simulink library "LIB_RespiratorSupervisor"  (R2018b)
settings: Solver=VariableStepAuto  StartTime=0.0  StopTime=10.0  RelTol=1e-3
undefined symbols (not defined in the file or in its folder): eSupervisorStates, tDelayMaxForRespiratorInit, tDelayMaxForTestMode, tMaxDebounceForCycleStop, tMinDebounceForTestStart
libraries: simulink x8, LIB_CycleControl x1
settings Model: Creator=BRAUL  LastModifiedBy=VITIE

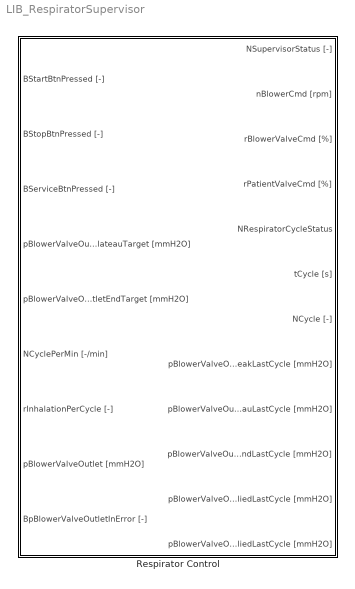
== system LIB_RespiratorSupervisor ==
  Respirator Control : Subsystem
      settings: AttributesFormatString=%<ReferenceBlock>

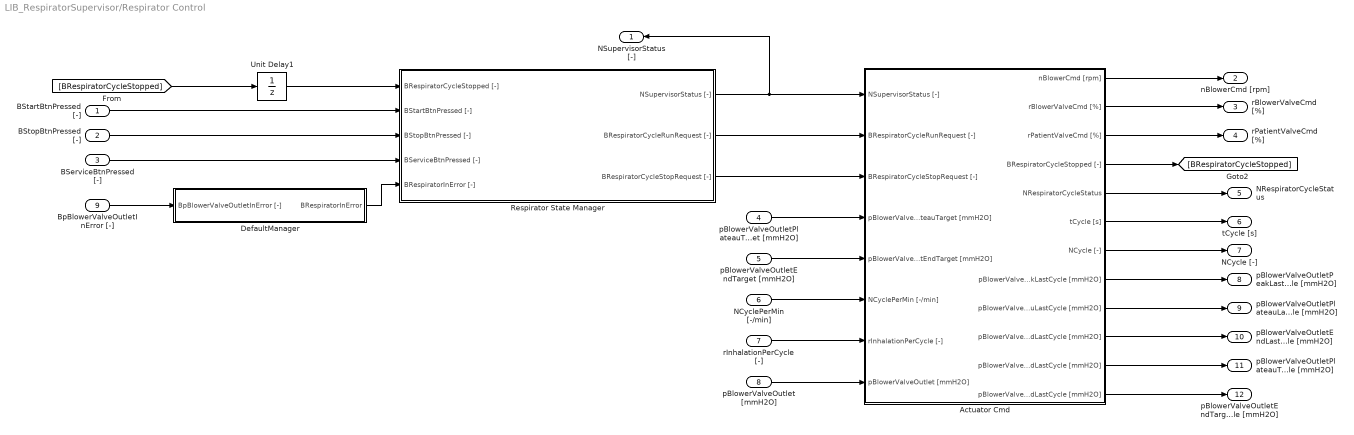
== system LIB_RespiratorSupervisor/Respirator Control ==
  BStartBtnPressed [-] : Inport  OutDataTypeStr=boolean
  BStopBtnPressed [-] : Inport  Port=2  OutDataTypeStr=boolean
  BServiceBtnPressed [-] : Inport  Port=3  OutDataTypeStr=boolean
  pBlowerValveOutletPlateauTarget [mmH2O] : Inport  Port=4  OutDataTypeStr=single
  pBlowerValveOutletEndTarget [mmH2O] : Inport  Port=5  OutDataTypeStr=single
  NCyclePerMin [-/min] : Inport  Port=6  OutDataTypeStr=single
  rInhalationPerCycle [-] : Inport  Port=7  OutDataTypeStr=single
  pBlowerValveOutlet [mmH2O] : Inport  Port=8  OutDataTypeStr=single
  BpBlowerValveOutletInError [-] : Inport  Port=9  OutDataTypeStr=boolean
  Actuator Cmd : Subsystem
  DefaultManager : Subsystem
  Respirator State Manager : Subsystem
  Unit Delay1 : UnitDelay  InitialCondition=false  SampleTime=-1
      settings: AttributesFormatString=%<InitialCondition>
  NSupervisorStatus [-] : Outport  OutDataTypeStr=Enum: eSupervisorStates  LockScale=on
  nBlowerCmd [rpm] : Outport  Port=2  OutDataTypeStr=single
  rBlowerValveCmd [%] : Outport  Port=3  OutDataTypeStr=single
  rPatientValveCmd [%] : Outport  Port=4  OutDataTypeStr=single
  NRespiratorCycleStatus : Outport  Port=5
  tCycle [s] : Outport  Port=6
  NCycle [-] : Outport  Port=7
  pBlowerValveOutletPeakLastCycle [mmH2O] : Outport  Port=8
  pBlowerValveOutletPlateauLastCycle [mmH2O] : Outport  Port=9  InitialOutput=0
  pBlowerValveOutletEndLastCycle [mmH2O] : Outport  Port=10
  pBlowerValveOutletPlateauTargetAppliedLastCycle [mmH2O] : Outport  Port=11
  pBlowerValveOutletEndTargetAppliedLastCycle [mmH2O] : Outport  Port=12
  wires:
  Actuator Cmd/7(NCycle [-]) -> NCycle [-]/1
  Actuator Cmd/8(pBlowerValveOutletPeakLastCycle [mmH2O]) -> pBlowerValveOutletPeakLastCycle [mmH2O]/1
  Actuator Cmd/12(pBlowerValveOutletEndTargetAppliedLastCycle [mmH2O]) -> pBlowerValveOutletEndTargetAppliedLastCycle [mmH2O]/1
  Actuator Cmd/10(pBlowerValveOutletEndLastCycle [mmH2O]) -> pBlowerValveOutletEndLastCycle [mmH2O]/1
  Actuator Cmd/11(pBlowerValveOutletPlateauTargetAppliedLastCycle [mmH2O]) -> pBlowerValveOutletPlateauTargetAppliedLastCycle [mmH2O]/1
  Actuator Cmd/9(pBlowerValveOutletPlateauLastCycle [mmH2O]) -> pBlowerValveOutletPlateauLastCycle [mmH2O]/1
  Actuator Cmd/5(NRespiratorCycleStatus) -> NRespiratorCycleStatus/1
  Actuator Cmd/6(tCycle [s]) -> tCycle [s]/1
  Respirator State Manager/1(NSupervisorStatus [-]) -> Actuator Cmd/1(NSupervisorStatus [-]), NSupervisorStatus [-]/1
  BpBlowerValveOutletInError [-]/1 -> DefaultManager/1(BpBlowerValveOutletInError [-])
  BServiceBtnPressed [-]/1 -> Respirator State Manager/4(BServiceBtnPressed [-])
  BStopBtnPressed [-]/1 -> Respirator State Manager/3(BStopBtnPressed [-])
  Unit Delay1/1 -> Respirator State Manager/1(BRespiratorCycleStopped [-])
  BStartBtnPressed [-]/1 -> Respirator State Manager/2(BStartBtnPressed [-])
  [BRespiratorCycleStopped] -> Unit Delay1/1
  Respirator State Manager/2(BRespiratorCycleRunRequest [-]) -> Actuator Cmd/2(BRespiratorCycleRunRequest [-])
  Respirator State Manager/3(BRespiratorCycleStopRequest [-]) -> Actuator Cmd/3(BRespiratorCycleStopRequest [-])
  pBlowerValveOutletPlateauTarget [mmH2O]/1 -> Actuator Cmd/4(pBlowerValveOutletPlateauTarget [mmH2O])
  pBlowerValveOutletEndTarget [mmH2O]/1 -> Actuator Cmd/5(pBlowerValveOutletEndTarget [mmH2O])
  NCyclePerMin [-/min]/1 -> Actuator Cmd/6(NCyclePerMin [-/min])
  rInhalationPerCycle [-]/1 -> Actuator Cmd/7(rInhalationPerCycle [-])
  Actuator Cmd/1(nBlowerCmd [rpm]) -> nBlowerCmd [rpm]/1
  Actuator Cmd/2(rBlowerValveCmd [%]) -> rBlowerValveCmd [%]/1
  Actuator Cmd/3(rPatientValveCmd [%]) -> rPatientValveCmd [%]/1
  Actuator Cmd/4(BRespiratorCycleStopped [-]) -> [BRespiratorCycleStopped]
  DefaultManager/1(BRespiratorInError) -> Respirator State Manager/5(BRespiratorInError [-])
  pBlowerValveOutlet [mmH2O]/1 -> Actuator Cmd/8(pBlowerValveOutlet [mmH2O])

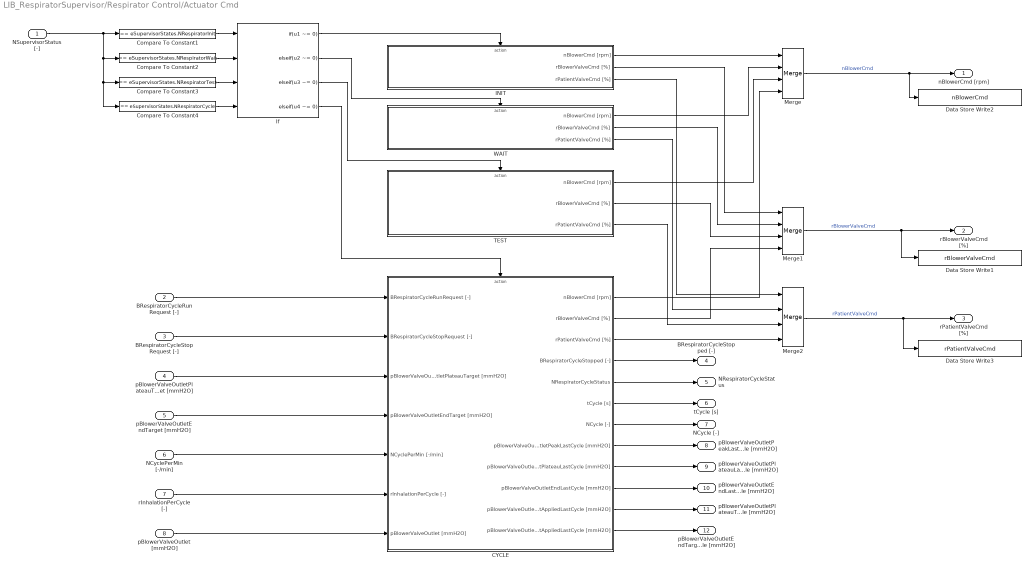
== system LIB_RespiratorSupervisor/Respirator Control/Actuator Cmd ==
  NSupervisorStatus [-] : Inport
  BRespiratorCycleRunRequest [-] : Inport  Port=2
  BRespiratorCycleStopRequest [-] : Inport  Port=3
  pBlowerValveOutletPlateauTarget [mmH2O] : Inport  Port=4  OutDataTypeStr=single
  pBlowerValveOutletEndTarget [mmH2O] : Inport  Port=5  OutDataTypeStr=single
  NCyclePerMin [-/min] : Inport  Port=6  OutDataTypeStr=single
  rInhalationPerCycle [-] : Inport  Port=7  OutDataTypeStr=single
  pBlowerValveOutlet [mmH2O] : Inport  Port=8  OutDataTypeStr=single
  CYCLE : Subsystem
  Compare To Constant1 : simulink/Logic and Bit Operations/Compare To Constant  relop===  const=eSupervisorStates.NRespiratorInit  OutDataTypeStr=boolean
  Compare To Constant2 : simulink/Logic and Bit Operations/Compare To Constant  relop===  const=eSupervisorStates.NRespiratorWait  OutDataTypeStr=boolean
  Compare To Constant3 : simulink/Logic and Bit Operations/Compare To Constant  relop===  const=eSupervisorStates.NRespiratorTest  OutDataTypeStr=boolean
  Compare To Constant4 : simulink/Logic and Bit Operations/Compare To Constant  relop===  const=eSupervisorStates.NRespiratorCycle  OutDataTypeStr=boolean
  Data Store Write1 : DataStoreWrite  DataStoreName=rBlowerValveCmd
  Data Store Write2 : DataStoreWrite  DataStoreName=nBlowerCmd
  Data Store Write3 : DataStoreWrite  DataStoreName=rPatientValveCmd
  INIT : Subsystem
  If : If  NumInputs=4  IfExpression=u1 ~= 0  ElseIfExpressions=u2 ~= 0,u3 ~= 0,u4 ~= 0  ShowElse=off
  Merge : Merge  Inputs=4  InitialOutput=0
  Merge1 : Merge  Inputs=4  InitialOutput=0
  Merge2 : Merge  Inputs=4  InitialOutput=0
  TEST : Subsystem
  WAIT : Subsystem
  nBlowerCmd [rpm] : Outport  OutDataTypeStr=single
  rBlowerValveCmd [%] : Outport  Port=2  OutDataTypeStr=single
  rPatientValveCmd [%] : Outport  Port=3  OutDataTypeStr=single
  BRespiratorCycleStopped [-] : Outport  Port=4
  NRespiratorCycleStatus : Outport  Port=5
  tCycle [s] : Outport  Port=6
  NCycle [-] : Outport  Port=7
  pBlowerValveOutletPeakLastCycle [mmH2O] : Outport  Port=8
  pBlowerValveOutletPlateauLastCycle [mmH2O] : Outport  Port=9  InitialOutput=0
  pBlowerValveOutletEndLastCycle [mmH2O] : Outport  Port=10
  pBlowerValveOutletPlateauTargetAppliedLastCycle [mmH2O] : Outport  Port=11
  pBlowerValveOutletEndTargetAppliedLastCycle [mmH2O] : Outport  Port=12
  wires:
  CYCLE/7(NCycle [-]) -> NCycle [-]/1
  CYCLE/10(pBlowerValveOutletEndLastCycle [mmH2O]) -> pBlowerValveOutletEndLastCycle [mmH2O]/1
  CYCLE/8(pBlowerValveOutletPeakLastCycle [mmH2O]) -> pBlowerValveOutletPeakLastCycle [mmH2O]/1
  CYCLE/12(pBlowerValveOutletEndTargetAppliedLastCycle [mmH2O]) -> pBlowerValveOutletEndTargetAppliedLastCycle [mmH2O]/1
  CYCLE/9(pBlowerValveOutletPlateauLastCycle [mmH2O]) -> pBlowerValveOutletPlateauLastCycle [mmH2O]/1
  CYCLE/11(pBlowerValveOutletPlateauTargetAppliedLastCycle [mmH2O]) -> pBlowerValveOutletPlateauTargetAppliedLastCycle [mmH2O]/1
  CYCLE/6(tCycle [s]) -> tCycle [s]/1
  CYCLE/5(NRespiratorCycleStatus) -> NRespiratorCycleStatus/1
  WAIT/3(rPatientValveCmd [%]) -> Merge2/2
  If/1 -> INIT/Action
  TEST/1(nBlowerCmd [rpm]) -> Merge/3
  Compare To Constant4/1 -> If/4
  Compare To Constant2/1 -> If/2
  NCyclePerMin [-/min]/1 -> CYCLE/5(NCyclePerMin [-/min])
  INIT/1(nBlowerCmd [rpm]) -> Merge/1
  INIT/2(rBlowerValveCmd [%]) -> Merge1/1
  NSupervisorStatus [-]/1 -> Compare To Constant4/1, Compare To Constant3/1, Compare To Constant2/1, Compare To Constant1/1
  Merge/1 -> nBlowerCmd [rpm]/1, Data Store Write2/1  "nBlowerCmd"
  CYCLE/3(rPatientValveCmd [%]) -> Merge2/4
  WAIT/2(rBlowerValveCmd [%]) -> Merge1/2
  rInhalationPerCycle [-]/1 -> CYCLE/6(rInhalationPerCycle [-])
  pBlowerValveOutletPlateauTarget [mmH2O]/1 -> CYCLE/3(pBlowerValveOutletPlateauTarget [mmH2O])
  If/2 -> WAIT/Action
  Compare To Constant3/1 -> If/3
  pBlowerValveOutlet [mmH2O]/1 -> CYCLE/7(pBlowerValveOutlet [mmH2O])
  Merge2/1 -> Data Store Write3/1, rPatientValveCmd [%]/1  "rPatientValveCmd"
  If/3 -> TEST/Action
  CYCLE/1(nBlowerCmd [rpm]) -> Merge/4
  If/4 -> CYCLE/Action
  TEST/3(rPatientValveCmd [%]) -> Merge2/3
  TEST/2(rBlowerValveCmd [%]) -> Merge1/3
  BRespiratorCycleStopRequest [-]/1 -> CYCLE/2(BRespiratorCycleStopRequest [-])
  pBlowerValveOutletEndTarget [mmH2O]/1 -> CYCLE/4(pBlowerValveOutletEndTarget [mmH2O])
  Compare To Constant1/1 -> If/1
  Merge1/1 -> rBlowerValveCmd [%]/1, Data Store Write1/1  "rBlowerValveCmd"
  CYCLE/2(rBlowerValveCmd [%]) -> Merge1/4
  WAIT/1(nBlowerCmd [rpm]) -> Merge/2
  BRespiratorCycleRunRequest [-]/1 -> CYCLE/1(BRespiratorCycleRunRequest [-])
  INIT/3(rPatientValveCmd [%]) -> Merge2/1
  CYCLE/4(BRespiratorCycleStopped [-]) -> BRespiratorCycleStopped [-]/1

== system LIB_RespiratorSupervisor/Respirator Control/DefaultManager ==
  BpBlowerValveOutletInError [-] : Inport  OutDataTypeStr=boolean
  Data Store Write2 : DataStoreWrite  DataStoreName=BRespiratorInError
  Unit Delay : UnitDelay  SampleTime=-1
  BRespiratorInError : Outport
  wires:
  BpBlowerValveOutletInError [-]/1 -> Unit Delay/1
  Unit Delay/1 -> BRespiratorInError/1, Data Store Write2/1  "BRespiratorInError"

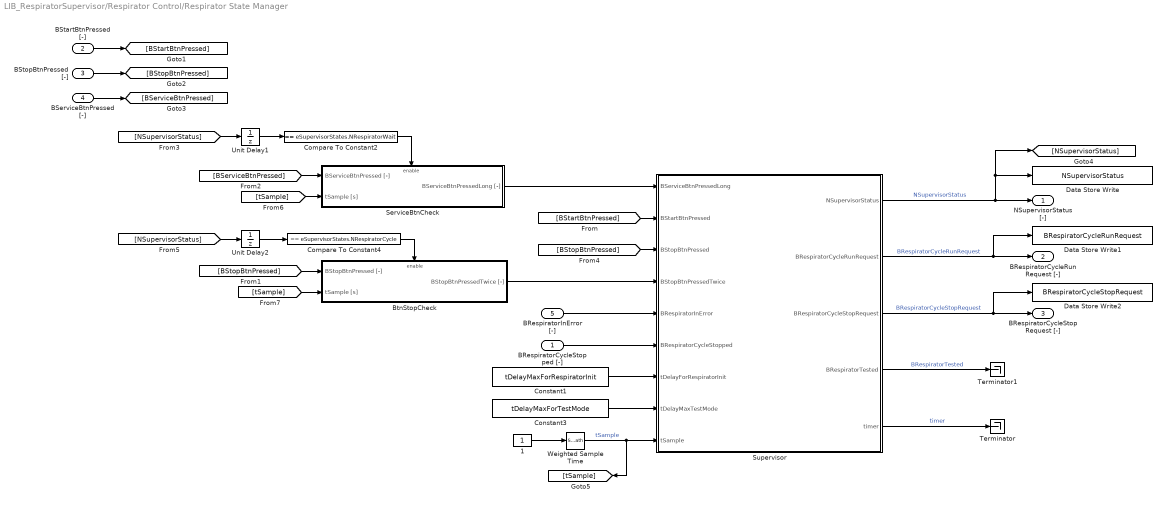
== system LIB_RespiratorSupervisor/Respirator Control/Respirator State Manager ==
  BRespiratorCycleStopped [-] : Inport
  BStartBtnPressed [-] : Inport  Port=2
  BStopBtnPressed [-] : Inport  Port=3
  BServiceBtnPressed [-] : Inport  Port=4
  BRespiratorInError [-] : Inport  Port=5
  1 : Constant  OutDataTypeStr=single
  BtnStopCheck : Subsystem
  Compare To Constant2 : simulink/Logic and Bit Operations/Compare To Constant  relop===  const=eSupervisorStates.NRespiratorWait  OutDataTypeStr=boolean
  Compare To Constant4 : simulink/Logic and Bit Operations/Compare To Constant  relop===  const=eSupervisorStates.NRespiratorCycle  OutDataTypeStr=boolean
  Constant1 : Constant  Value=tDelayMaxForRespiratorInit  OutDataTypeStr=single
  Constant3 : Constant  Value=tDelayMaxForTestMode  OutDataTypeStr=single
  Data Store Write : DataStoreWrite  DataStoreName=NSupervisorStatus
  Data Store Write1 : DataStoreWrite  DataStoreName=BRespiratorCycleRunRequest
  Data Store Write2 : DataStoreWrite  DataStoreName=BRespiratorCycleStopRequest
  ServiceBtnCheck : Subsystem
  Supervisor : Stateflow chart  TreatAsAtomicUnit=on
  Terminator : Terminator
  Terminator1 : Terminator
  Unit Delay1 : UnitDelay  InitialCondition=eSupervisorStates.NRespiratorInit  SampleTime=-1
      settings: AttributesFormatString=%<InitialCondition>
  Unit Delay2 : UnitDelay  InitialCondition=eSupervisorStates.NRespiratorInit  SampleTime=-1
      settings: AttributesFormatString=%<InitialCondition>
  Weighted Sample Time : SampleTimeMath  TsampMathOp=Ts Only  OutDataTypeStr=Inherit: Inherit via back propagation
  NSupervisorStatus [-] : Outport
  BRespiratorCycleRunRequest [-] : Outport  Port=2
  BRespiratorCycleStopRequest [-] : Outport  Port=3
  wires:
  Weighted Sample Time/1 -> [tSample], Supervisor/9(tSample)  "tSample"
  1/1 -> Weighted Sample Time/1
  Supervisor/1(NSupervisorStatus) -> [NSupervisorStatus], Data Store Write/1, NSupervisorStatus [-]/1  "NSupervisorStatus"
  Supervisor/5(timer) -> Terminator/1  "timer"
  Supervisor/4(BRespiratorTested) -> Terminator1/1  "BRespiratorTested"
  BStartBtnPressed [-]/1 -> [BStartBtnPressed]
  BStopBtnPressed [-]/1 -> [BStopBtnPressed]
  BServiceBtnPressed [-]/1 -> [BServiceBtnPressed]
  Supervisor/2(BRespiratorCycleRunRequest) -> BRespiratorCycleRunRequest [-]/1, Data Store Write1/1  "BRespiratorCycleRunRequest"
  Supervisor/3(BRespiratorCycleStopRequest) -> BRespiratorCycleStopRequest [-]/1, Data Store Write2/1  "BRespiratorCycleStopRequest"
  Constant3/1 -> Supervisor/8(tDelayMaxTestMode)
  Constant1/1 -> Supervisor/7(tDelayForRespiratorInit)
  [BStartBtnPressed] -> Supervisor/2(BStartBtnPressed)
  BRespiratorCycleStopped [-]/1 -> Supervisor/6(BRespiratorCycleStopped)
  [BStopBtnPressed] -> Supervisor/3(BStopBtnPressed)
  BtnStopCheck/1(BStopBtnPressedTwice [-]) -> Supervisor/4(BStopBtnPressedTwice)
  ServiceBtnCheck/1(BServiceBtnPressedLong [-]) -> Supervisor/1(BServiceBtnPressedLong)
  [BStopBtnPressed] -> BtnStopCheck/1(BStopBtnPressed [-])
  [BServiceBtnPressed] -> ServiceBtnCheck/1(BServiceBtnPressed [-])
  Compare To Constant2/1 -> ServiceBtnCheck/Enable
  Compare To Constant4/1 -> BtnStopCheck/Enable
  [NSupervisorStatus] -> Unit Delay1/1
  [NSupervisorStatus] -> Unit Delay2/1
  Unit Delay1/1 -> Compare To Constant2/1
  Unit Delay2/1 -> Compare To Constant4/1
  [tSample] -> ServiceBtnCheck/2(tSample [s])
  [tSample] -> BtnStopCheck/2(tSample [s])
  BRespiratorInError [-]/1 -> Supervisor/5(BRespiratorInError)

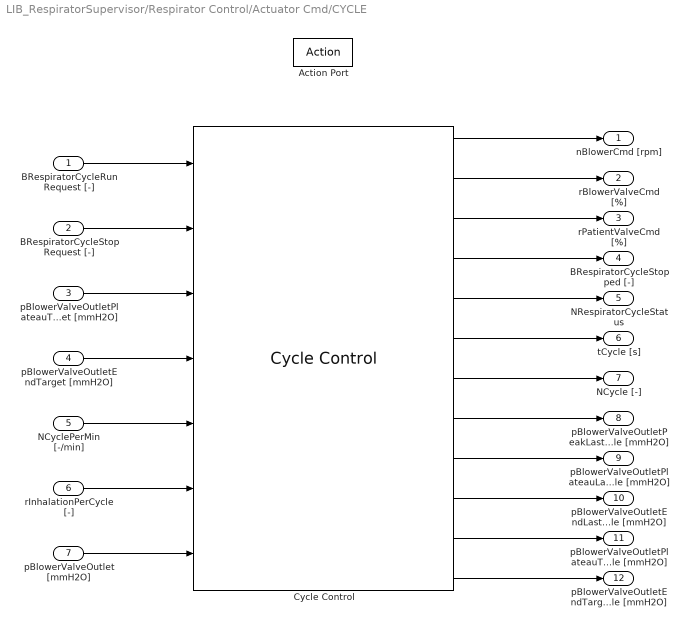
== system LIB_RespiratorSupervisor/Respirator Control/Actuator Cmd/CYCLE ==
  BRespiratorCycleRunRequest [-] : Inport
  BRespiratorCycleStopRequest [-] : Inport  Port=2
  pBlowerValveOutletPlateauTarget [mmH2O] : Inport  Port=3  OutDataTypeStr=single
  pBlowerValveOutletEndTarget [mmH2O] : Inport  Port=4  OutDataTypeStr=single
  NCyclePerMin [-/min] : Inport  Port=5  OutDataTypeStr=single
  rInhalationPerCycle [-] : Inport  Port=6  OutDataTypeStr=single
  pBlowerValveOutlet [mmH2O] : Inport  Port=7  OutDataTypeStr=single
  Action Port : ActionPort
  Cycle Control : LIB_CycleControl/Cycle Control  SystemSampleTime=-1
      settings: AttributesFormatString=%<ReferenceBlock>
  nBlowerCmd [rpm] : Outport  OutDataTypeStr=single
  rBlowerValveCmd [%] : Outport  Port=2  OutDataTypeStr=single
  rPatientValveCmd [%] : Outport  Port=3  OutDataTypeStr=single
  BRespiratorCycleStopped [-] : Outport  Port=4  InitialOutput=0
  NRespiratorCycleStatus : Outport  Port=5
  tCycle [s] : Outport  Port=6
  NCycle [-] : Outport  Port=7
  pBlowerValveOutletPeakLastCycle [mmH2O] : Outport  Port=8
  pBlowerValveOutletPlateauLastCycle [mmH2O] : Outport  Port=9  InitialOutput=0
  pBlowerValveOutletEndLastCycle [mmH2O] : Outport  Port=10
  pBlowerValveOutletPlateauTargetAppliedLastCycle [mmH2O] : Outport  Port=11
  pBlowerValveOutletEndTargetAppliedLastCycle [mmH2O] : Outport  Port=12
  wires:
  Cycle Control/7 -> NCycle [-]/1
  Cycle Control/9 -> pBlowerValveOutletPlateauLastCycle [mmH2O]/1
  Cycle Control/12 -> pBlowerValveOutletEndTargetAppliedLastCycle [mmH2O]/1
  Cycle Control/8 -> pBlowerValveOutletPeakLastCycle [mmH2O]/1
  Cycle Control/11 -> pBlowerValveOutletPlateauTargetAppliedLastCycle [mmH2O]/1
  Cycle Control/10 -> pBlowerValveOutletEndLastCycle [mmH2O]/1
  Cycle Control/6 -> tCycle [s]/1
  Cycle Control/5 -> NRespiratorCycleStatus/1
  rInhalationPerCycle [-]/1 -> Cycle Control/6
  pBlowerValveOutlet [mmH2O]/1 -> Cycle Control/7
  pBlowerValveOutletPlateauTarget [mmH2O]/1 -> Cycle Control/3
  pBlowerValveOutletEndTarget [mmH2O]/1 -> Cycle Control/4
  NCyclePerMin [-/min]/1 -> Cycle Control/5
  Cycle Control/3 -> rPatientValveCmd [%]/1
  Cycle Control/1 -> nBlowerCmd [rpm]/1
  Cycle Control/2 -> rBlowerValveCmd [%]/1
  Cycle Control/4 -> BRespiratorCycleStopped [-]/1
  BRespiratorCycleStopRequest [-]/1 -> Cycle Control/2
  BRespiratorCycleRunRequest [-]/1 -> Cycle Control/1

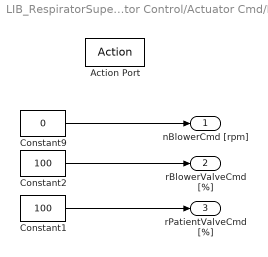
== system LIB_RespiratorSupervisor/Respirator Control/Actuator Cmd/INIT ==
  Action Port : ActionPort
  Constant1 : Constant  Value=100  OutDataTypeStr=Inherit: Inherit via back propagation
  Constant2 : Constant  Value=100  OutDataTypeStr=Inherit: Inherit via back propagation
  Constant9 : Constant  Value=0  OutDataTypeStr=single
  nBlowerCmd [rpm] : Outport
  rBlowerValveCmd [%] : Outport  Port=2
  rPatientValveCmd [%] : Outport  Port=3
  wires:
  Constant9/1 -> nBlowerCmd [rpm]/1
  Constant1/1 -> rPatientValveCmd [%]/1
  Constant2/1 -> rBlowerValveCmd [%]/1

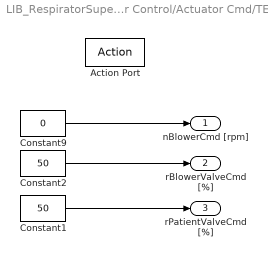
== system LIB_RespiratorSupervisor/Respirator Control/Actuator Cmd/TEST ==
  Action Port : ActionPort
  Constant1 : Constant  Value=50  OutDataTypeStr=Inherit: Inherit via back propagation
  Constant2 : Constant  Value=50  OutDataTypeStr=Inherit: Inherit via back propagation
  Constant9 : Constant  Value=0  OutDataTypeStr=single
  nBlowerCmd [rpm] : Outport
  rBlowerValveCmd [%] : Outport  Port=2
  rPatientValveCmd [%] : Outport  Port=3
  wires:
  Constant9/1 -> nBlowerCmd [rpm]/1
  Constant1/1 -> rPatientValveCmd [%]/1
  Constant2/1 -> rBlowerValveCmd [%]/1

== system LIB_RespiratorSupervisor/Respirator Control/Actuator Cmd/WAIT ==
  Action Port : ActionPort
  Constant1 : Constant  Value=100  OutDataTypeStr=Inherit: Inherit via back propagation
  Constant2 : Constant  Value=0  OutDataTypeStr=Inherit: Inherit via back propagation
  Constant9 : Constant  Value=0  OutDataTypeStr=single
  nBlowerCmd [rpm] : Outport
  rBlowerValveCmd [%] : Outport  Port=2
  rPatientValveCmd [%] : Outport  Port=3
  wires:
  Constant2/1 -> rBlowerValveCmd [%]/1
  Constant1/1 -> rPatientValveCmd [%]/1
  Constant9/1 -> nBlowerCmd [rpm]/1

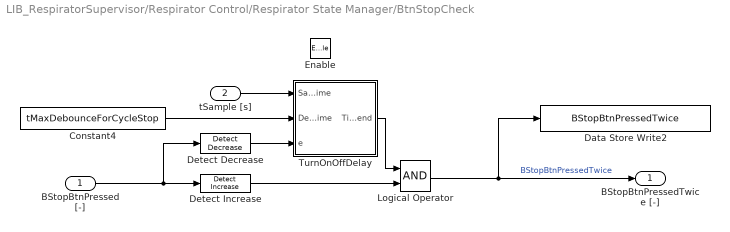
== system LIB_RespiratorSupervisor/Respirator Control/Respirator State Manager/BtnStopCheck ==
  BStopBtnPressed [-] : Inport
  tSample [s] : Inport  Port=2
  Enable : EnablePort
  Constant4 : Constant  Value=tMaxDebounceForCycleStop  OutDataTypeStr=single
  Data Store Write2 : DataStoreWrite  DataStoreName=BStopBtnPressedTwice
  Detect Decrease : simulink/Logic and Bit Operations/Detect Decrease  vinit=0.0  OutDataTypeStr=boolean
  Detect Increase : simulink/Logic and Bit Operations/Detect Increase  vinit=0.0  OutDataTypeStr=boolean
  Logical Operator : Logic  AllPortsSameDT=off  OutDataTypeStr=boolean
  TurnOnOffDelay : Subsystem  mask(TurnOn/OffDelay){DelayType=Turn Off Delay, OutDataType=boolean}
      mask prompts: DelayType "Delay Type"; OutDataType "Out Data Type"
      mask help: Bloc de confirmation de montée/chute si e est/n'est plus vrai pendant une durée T (en secondes)
      mask init:
      | LogicBlocks=find_system(gcbh,'LookUnderMasks','all','FollowLinks','On','SearchDepth','1','BlockType','Logic');
      | DetectionBlock=find_system(gcbh,'LookUnderMasks','all','FollowLinks','On','SearchDepth','1','MaskType','DETECTIONFRONT');
      | if DelayType==1
      | set_param(LogicBlocks(1),'Operator','AND');
      | set_param(LogicBlocks(2),'Operator','AND');
      | set_param(DetectionBlock,'FrontType','Rising');
      | FrontIconY=[0.2 0.2 0.6 0.6];
      | else
      | set_param(LogicBlocks(1),'Operator','OR')
      | set_param(LogicBlocks(2),'Operator','NOT');
      | set_param(DetectionBlock,'FrontType','Falling');
      | FrontIconY=[0.6 0.6 0.2 0.2];
      | end
      | 
      | ConversionBlock=find_system(gcbh,'LookUnderMasks','all','FollowLinks','On','SearchDepth','1','BlockType','DataTypeConversion');
      | DataTypeOptionsStr=[{'Inherit: Inherit via back propagation'},{'double'},{'single'},{'int8'},{'uint8'},{'int16'},{'uint16'},{'int32'},{'uint32'},{'boolean'},{'fixdt(1,16)'},{'fixdt(1,16,0)'},{'fixdt(1,16,2^0,0)'},{'Enum: <class name>'},{'<data type expression>'}]
      | set_param(ConversionBlock,'OutDataTypeStr',DataTypeOptionsStr{OutDataType});
      settings: AttributesFormatString=%<StaticLinkStatus>
      mask TypeOptions DelayType: Turn On Delay | Turn Off Delay
      mask TypeOptions OutDataType: Inherit: Inherit via back propagation | double | single | int8 | uint8 | int16 | uint16 | int32 | uint32 | boolean | fixdt(1,16) | fixdt(1,16,0) | fixdt(1,16,2^0,0) | Enum: <class name> | <data type expression>
      mask Display:
      | plot([0.3 0.6 0.6 0.9], FrontIconY);
      | port_label('input',2,'T [s]')
      | port_label('input',3,'e')
      | port_label('input',1,'Ts [s]')
      | text(0.4,0.4, 'T');
  BStopBtnPressedTwice [-] : Outport  OutputWhenDisabled=reset  InitialOutput=0
  wires:
  Logical Operator/1 -> BStopBtnPressedTwice [-]/1, Data Store Write2/1  "BStopBtnPressedTwice"
  BStopBtnPressed [-]/1 -> Detect Decrease/1, Detect Increase/1
  Detect Increase/1 -> Logical Operator/2
  Detect Decrease/1 -> TurnOnOffDelay/3(e)
  Constant4/1 -> TurnOnOffDelay/2(DelayTime)
  TurnOnOffDelay/1(Timer_end) -> Logical Operator/1
  tSample [s]/1 -> TurnOnOffDelay/1(SampleTime)

== system LIB_RespiratorSupervisor/Respirator Control/Respirator State Manager/ServiceBtnCheck ==
  BServiceBtnPressed [-] : Inport
  tSample [s] : Inport  Port=2
  Enable : EnablePort
  Constant2 : Constant  Value=tMinDebounceForTestStart  OutDataTypeStr=single
  Data Store Write2 : DataStoreWrite  DataStoreName=BServiceBtnPressedLong
  TurnOnOffDelay : Subsystem  mask(TurnOn/OffDelay){DelayType=Turn On Delay, OutDataType=boolean}
      mask prompts: DelayType "Delay Type"; OutDataType "Out Data Type"
      mask help: Bloc de confirmation de montée/chute si e est/n'est plus vrai pendant une durée T (en secondes)
      mask init: same as LIB_RespiratorSupervisor/Respirator Control/Respirator State Manager/BtnStopCheck/TurnOnOffDelay
      settings: AttributesFormatString=%<StaticLinkStatus>
      mask TypeOptions DelayType: Turn On Delay | Turn Off Delay
      mask TypeOptions OutDataType: Inherit: Inherit via back propagation | double | single | int8 | uint8 | int16 | uint16 | int32 | uint32 | boolean | fixdt(1,16) | fixdt(1,16,0) | fixdt(1,16,2^0,0) | Enum: <class name> | <data type expression>
      mask Display:
      | plot([0.3 0.6 0.6 0.9], FrontIconY);
      | port_label('input',2,'T [s]')
      | port_label('input',3,'e')
      | port_label('input',1,'Ts [s]')
      | text(0.4,0.4, 'T');
  BServiceBtnPressedLong [-] : Outport  OutputWhenDisabled=reset  InitialOutput=0
  wires:
  TurnOnOffDelay/1(Timer_end) -> BServiceBtnPressedLong [-]/1, Data Store Write2/1  "BServiceBtnPressedLong"
  Constant2/1 -> TurnOnOffDelay/2(DelayTime)
  BServiceBtnPressed [-]/1 -> TurnOnOffDelay/3(e)
  tSample [s]/1 -> TurnOnOffDelay/1(SampleTime)

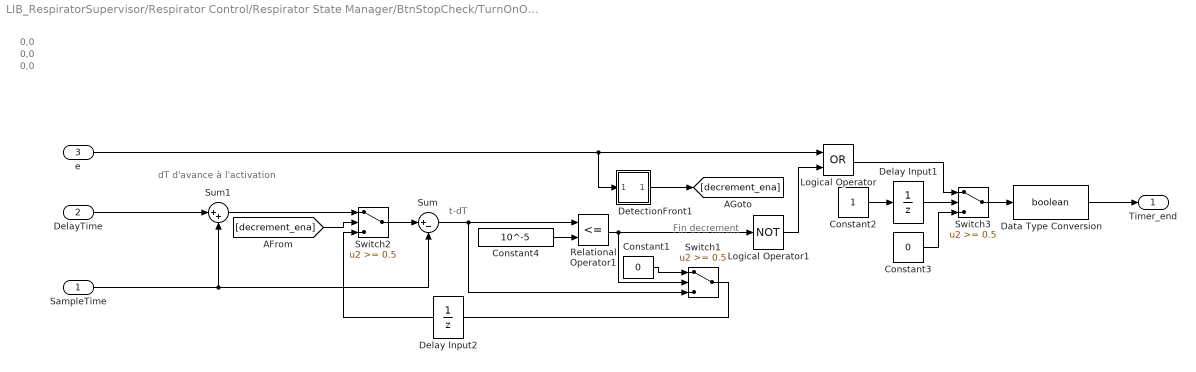
== system LIB_RespiratorSupervisor/Respirator Control/Respirator State Manager/BtnStopCheck/TurnOnOffDelay ==
  note: 0,0
  note: 0,0
  note: 0,0
  note: 0,0
  note: 0,0
  note: 0,0
  note: 0,0
  note: Fin decrement
  note: t-dT
  note: dT d'avance à l'activation
  SampleTime : Inport
  DelayTime : Inport  Port=2
  e : Inport  Port=3
  Constant1 : Constant  Value=0
  Constant2 : Constant
  Constant3 : Constant  Value=0
  Constant4 : Constant  Tag=AM,Constant,0,1,Value;CMP,Value;  Value=10^-5
  Data Type Conversion : DataTypeConversion  OutDataTypeStr=boolean
  Delay Input1 : UnitDelay  Description=\nStore in Global RAM  SampleTime=-1
  Delay Input2 : UnitDelay  Description=\nStore in Global RAM  SampleTime=-1
  DetectionFront1 : Subsystem  mask(DETECTIONFRONT){FrontType=Falling, InitialValue=0}
      mask prompts: FrontType "Type de front :"; InitialValue "Condition initiale :"
      mask help:
      | Detecte un front sur un signal binaire :
      | - descendant (Falling)
      | - montant (Rising)
      | - les deux (Either).
      mask init:
      | if (FrontType==1);x=[0 1 1 2];y=[0 0 1 1];
      | elseif (FrontType==2);x=[0 1 1 2];y=[1 1 0 0];
      | else;x=[0 1 1 2;3 4 4 5]';y=[0 0 1 1;1 1 0 0]';end;
      mask TypeOptions FrontType: Rising | Falling | Either
      mask Display: plot(x,y)
  Logical Operator : Logic  Operator=OR  AllPortsSameDT=off  OutDataTypeStr=boolean
  Logical Operator1 : Logic  Operator=NOT  Inputs=1  AllPortsSameDT=off  OutDataTypeStr=boolean
  Relational Operator1 : RelationalOperator  Operator=<=  ZeroCross=off  RndMeth=Nearest
  Sum : Sum  Inputs=|+-
  Sum1 : Sum  Inputs=|++
  Switch1 : Switch  Tag=GEN,Threshold;AM,Switch,2,1;CMP,Threshold;  Threshold=0.5  SaturateOnIntegerOverflow=on
  Switch2 : Switch  Tag=GEN,Threshold;AM,Switch,2,1;CMP,Threshold;  Threshold=0.5  SaturateOnIntegerOverflow=on
  Switch3 : Switch  Tag=GEN,Threshold;AM,Switch,2,1;CMP,Threshold;  Threshold=0.5  SaturateOnIntegerOverflow=on
  Timer_end : Outport
  wires:
  Data Type Conversion/1 -> Timer_end/1
  Constant3/1 -> Switch3/3
  Logical Operator/1 -> Switch3/1
  Switch3/1 -> Data Type Conversion/1
  Delay Input1/1 -> Switch3/2
  Constant2/1 -> Delay Input1/1
  Constant4/1 -> Relational Operator1/2
  DetectionFront1/1(Front) -> [decrement_ena]
  Switch1/1 -> Delay Input2/1
  Constant1/1 -> Switch1/1
  Delay Input2/1 -> Switch2/3
  Switch2/1 -> Sum/1
  Sum1/1 -> Switch2/1
  [decrement_ena] -> Switch2/2
  Relational Operator1/1 -> Switch1/2, Logical Operator1/1
  Sum/1 -> Switch1/3, Relational Operator1/1
  DelayTime/1 -> Sum1/1
  SampleTime/1 -> Sum/2, Sum1/2
  e/1 -> DetectionFront1/1(Entree), Logical Operator/1
  Logical Operator1/1 -> Logical Operator/2

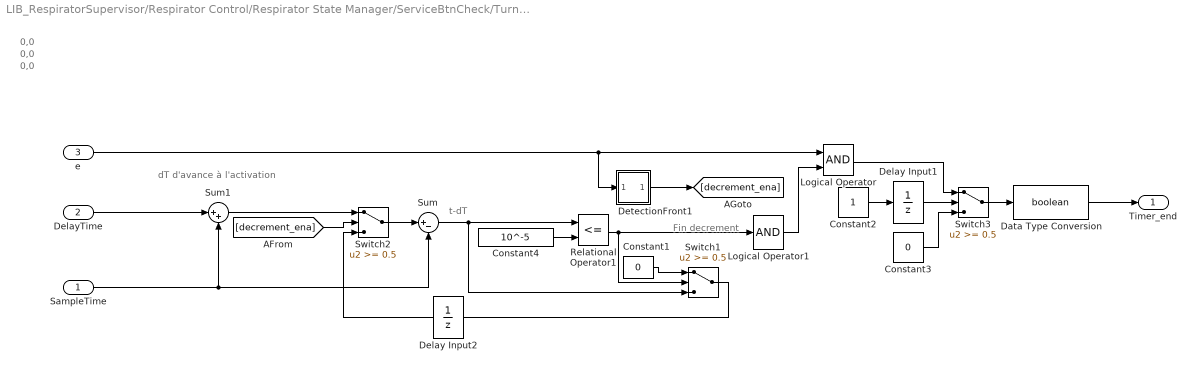
== system LIB_RespiratorSupervisor/Respirator Control/Respirator State Manager/ServiceBtnCheck/TurnOnOffDelay ==
  note: 0,0
  note: 0,0
  note: 0,0
  note: 0,0
  note: 0,0
  note: 0,0
  note: 0,0
  note: Fin decrement
  note: t-dT
  note: dT d'avance à l'activation
  SampleTime : Inport
  DelayTime : Inport  Port=2
  e : Inport  Port=3
  Constant1 : Constant  Value=0
  Constant2 : Constant
  Constant3 : Constant  Value=0
  Constant4 : Constant  Tag=AM,Constant,0,1,Value;CMP,Value;  Value=10^-5
  Data Type Conversion : DataTypeConversion  OutDataTypeStr=boolean
  Delay Input1 : UnitDelay  Description=\nStore in Global RAM  SampleTime=-1
  Delay Input2 : UnitDelay  Description=\nStore in Global RAM  SampleTime=-1
  DetectionFront1 : Subsystem  mask(DETECTIONFRONT){FrontType=Rising, InitialValue=0}
      mask prompts: FrontType "Type de front :"; InitialValue "Condition initiale :"
      mask help:
      | Detecte un front sur un signal binaire :
      | - descendant (Falling)
      | - montant (Rising)
      | - les deux (Either).
      mask init:
      | if (FrontType==1);x=[0 1 1 2];y=[0 0 1 1];
      | elseif (FrontType==2);x=[0 1 1 2];y=[1 1 0 0];
      | else;x=[0 1 1 2;3 4 4 5]';y=[0 0 1 1;1 1 0 0]';end;
      mask TypeOptions FrontType: Rising | Falling | Either
      mask Display: plot(x,y)
  Logical Operator : Logic  AllPortsSameDT=off  OutDataTypeStr=boolean
  Logical Operator1 : Logic  Inputs=1  AllPortsSameDT=off  OutDataTypeStr=boolean
  Relational Operator1 : RelationalOperator  Operator=<=  ZeroCross=off  RndMeth=Nearest
  Sum : Sum  Inputs=|+-
  Sum1 : Sum  Inputs=|++
  Switch1 : Switch  Tag=GEN,Threshold;AM,Switch,2,1;CMP,Threshold;  Threshold=0.5  SaturateOnIntegerOverflow=on
  Switch2 : Switch  Tag=GEN,Threshold;AM,Switch,2,1;CMP,Threshold;  Threshold=0.5  SaturateOnIntegerOverflow=on
  Switch3 : Switch  Tag=GEN,Threshold;AM,Switch,2,1;CMP,Threshold;  Threshold=0.5  SaturateOnIntegerOverflow=on
  Timer_end : Outport
  wires:
  Data Type Conversion/1 -> Timer_end/1
  Constant3/1 -> Switch3/3
  Logical Operator/1 -> Switch3/1
  Switch3/1 -> Data Type Conversion/1
  Delay Input1/1 -> Switch3/2
  Constant2/1 -> Delay Input1/1
  Constant4/1 -> Relational Operator1/2
  DetectionFront1/1(Front) -> [decrement_ena]
  Switch1/1 -> Delay Input2/1
  Constant1/1 -> Switch1/1
  Delay Input2/1 -> Switch2/3
  Switch2/1 -> Sum/1
  Sum1/1 -> Switch2/1
  [decrement_ena] -> Switch2/2
  Relational Operator1/1 -> Switch1/2, Logical Operator1/1
  Sum/1 -> Switch1/3, Relational Operator1/1
  DelayTime/1 -> Sum1/1
  SampleTime/1 -> Sum/2, Sum1/2
  e/1 -> DetectionFront1/1(Entree), Logical Operator/1
  Logical Operator1/1 -> Logical Operator/2

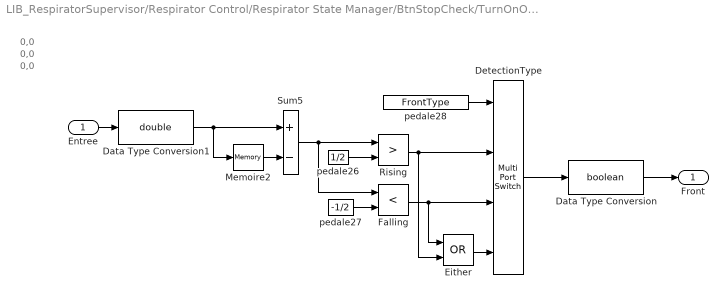
== system LIB_RespiratorSupervisor/Respirator Control/Respirator State Manager/BtnStopCheck/TurnOnOffDelay/DetectionFront1 ==
  note: 0,0
  note: 0,0
  note: 0,0
  note: 0,0
  note: 0,0
  note: 0,0
  note: 0,0
  Entree : Inport
  Data Type Conversion : DataTypeConversion  OutDataTypeStr=boolean
  Data Type Conversion1 : DataTypeConversion  OutDataTypeStr=double
  DetectionType : MultiPortSwitch  SaturateOnIntegerOverflow=on  InputSameDT=on
  Either : Logic  Operator=OR
  Falling : RelationalOperator  Operator=<  RndMeth=Nearest  InputSameDT=on
  Memoire2 : Memory  InitialCondition=InitialValue  InheritSampleTime=on
  Rising : RelationalOperator  Operator=>  RndMeth=Nearest  InputSameDT=on
  Sum5 : Sum  Inputs=+-  SaturateOnIntegerOverflow=on  InputSameDT=on  OutDataTypeStr=Inherit: Same as first input
  pedale26 : Constant  Value=1/2
  pedale27 : Constant  Value=-1/2
  pedale28 : Constant  Value=FrontType
  Front : Outport  InitialOutput=0
  wires:
  Memoire2/1 -> Sum5/2
  Entree/1 -> Data Type Conversion1/1
  Sum5/1 -> Rising/1, Falling/1
  DetectionType/1 -> Data Type Conversion/1
  Either/1 -> DetectionType/4
  Falling/1 -> DetectionType/3, Either/1
  pedale26/1 -> Rising/2
  pedale27/1 -> Falling/2
  Rising/1 -> DetectionType/2, Either/2
  pedale28/1 -> DetectionType/1
  Data Type Conversion/1 -> Front/1
  Data Type Conversion1/1 -> Memoire2/1, Sum5/1

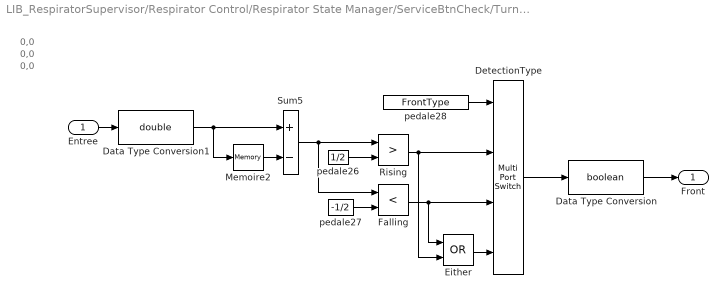
== system LIB_RespiratorSupervisor/Respirator Control/Respirator State Manager/ServiceBtnCheck/TurnOnOffDelay/DetectionFront1 ==
  note: 0,0
  note: 0,0
  note: 0,0
  note: 0,0
  note: 0,0
  note: 0,0
  note: 0,0
  Entree : Inport
  Data Type Conversion : DataTypeConversion  OutDataTypeStr=boolean
  Data Type Conversion1 : DataTypeConversion  OutDataTypeStr=double
  DetectionType : MultiPortSwitch  SaturateOnIntegerOverflow=on  InputSameDT=on
  Either : Logic  Operator=OR
  Falling : RelationalOperator  Operator=<  RndMeth=Nearest  InputSameDT=on
  Memoire2 : Memory  InitialCondition=InitialValue  InheritSampleTime=on
  Rising : RelationalOperator  Operator=>  RndMeth=Nearest  InputSameDT=on
  Sum5 : Sum  Inputs=+-  SaturateOnIntegerOverflow=on  InputSameDT=on  OutDataTypeStr=Inherit: Same as first input
  pedale26 : Constant  Value=1/2
  pedale27 : Constant  Value=-1/2
  pedale28 : Constant  Value=FrontType
  Front : Outport  InitialOutput=0
  wires:
  Memoire2/1 -> Sum5/2
  Entree/1 -> Data Type Conversion1/1
  Sum5/1 -> Rising/1, Falling/1
  DetectionType/1 -> Data Type Conversion/1
  Either/1 -> DetectionType/4
  Falling/1 -> DetectionType/3, Either/1
  pedale26/1 -> Rising/2
  pedale27/1 -> Falling/2
  Rising/1 -> DetectionType/2, Either/2
  pedale28/1 -> DetectionType/1
  Data Type Conversion/1 -> Front/1
  Data Type Conversion1/1 -> Memoire2/1, Sum5/1

== stateflow chart LIB_RespiratorSupervisor/Respirator Control/Respirator State Manager/Supervisor ==
  state SUPERVISOR
    entry:
    BRespiratorTested=true;
    BRespiratorCycleRunRequest=false;
    BRespiratorCycleStopRequest=false;
    state INIT
      entry :
      timer=tSample;
      NSupervisorStatus...
      =eSupervisorStates.NRespiratorInit;
      during: timer=timer+tSample;
    state WAIT
      entry:
      NSupervisorStatus...
      =eSupervisorStates.NRespiratorWait;
    state TEST_MODE
      entry: NSupervisorStatus...
      =eSupervisorStates.NRespiratorTest;
      timer=tSample;
      BRespiratorTested=false;
      during: timer=timer+tSample;
    state CYCLE_MODE
      entry:
      NSupervisorStatus...
      =eSupervisorStates.NRespiratorCycle;
    (default) -> INIT
    INIT -> WAIT : [timer>tDelayForRespiratorInit-tSample/2]
    WAIT -> TEST_MODE [order 1] : [BServiceBtnPressedLong]
    TEST_MODE -> WAIT : [timer>tDelayMaxTestMode-tSample/2]
        | {BRespiratorTested=true;}
    WAIT -> CYCLE_MODE [order 2] : [(BStartBtnPressed)&&...
        | (~BStopBtnPressed)&&...
        | (~BRespiratorInError)]
        | {BRespiratorCycleRunRequest=true;}
    CYCLE_MODE -> WAIT [order 2] : [BRespiratorCycleStopRequest&&...
        | BRespiratorCycleStopped]
        | {BRespiratorCycleStopRequest=false;}
    CYCLE_MODE -> CYCLE_MODE [order 1] : [BStopBtnPressedTwice...
        | ||BRespiratorInError]
        | {BRespiratorCycleRunRequest=false;
        | BRespiratorCycleStopRequest=true;}
  data: NSupervisorStatus output Enum: eSupervisorStates =eSupervisorStates.NRespiratorInit; BRespiratorCycleRunRequest output boolean [0..1] =true; BRespiratorCycleStopRequest output boolean [0..1] =true; BServiceBtnPressedLong input [0..1]; BStartBtnPressed input [0..1]; BStopBtnPressed input; BStopBtnPressedTwice input [0..1]; BRespiratorInError input [0..1]; BRespiratorCycleStopped input [0..1]; tDelayForRespiratorInit input [0..65535]; tDelayMaxTestMode input [0..65535]; tSample input [0..65535]; BRespiratorTested output boolean [0..1] =true; timer output single [0..65535]
